simulink library "albedo_lib"  (Simulink 6.3)
undefined symbols (not defined in the file or in its folder): albedo_path, albedo_wrapper, filesep, mean_refl, ss_proj
libraries: simulink x1
settings Model: LastModifiedBy=danji  StrictBusMsg=None

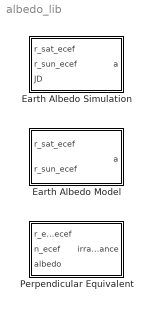
== system albedo_lib ==
  Earth Albedo Model : Subsystem  TreatAsAtomicUnit=on  mask(Earth Albedo Model){refldata=mean_refl, redfac=4, Ts=-1, enable=on}
      mask prompts: refldata "Reflectivity Data (REFL Struct):"; redfac "Reduction factor:"; Ts "Sample Time (-1 for inherited):"
      mask help: Calculcates the Earth albedo from satellite and Sun positions and static reflectivity data.
      mask init:
      | global sy;
      | global sx;
      | sy = floor(180/redfac);
      | sx = floor(288/redfac);
      mask Help:
      | <b>Input</b><br>
      | Sat: Vector to satellite in ECEF [m].<br>
      | Sun: Vector to the Sun in ECEF [m].<p>
      | <b>Parameters</b><br>
      | Reflectivity Data (REFL Struct): TOMS Reflectivity data [E.U].<br>
      | Reduction factor: Reduce data resolution by this factor.<br>
      | Sample Time (-1 for inherited): Sample Time [s]. The block cannot inherit continuous sample time.<br>
      | Enable: Enable or disable albedo calculation.<p>
      | <b>Output</b><br>
      | Albedo: Fraction of solar irradiance received on the satellite. The incoming solar irradiance is 1366.5 W/m^2.<p>
      mask CallbackString: |||enable = strcmp(get_param(gcb,'enable'),'on');
      mask Display:
      | image(imread('private/albedoicon.png'));
      | port_label('output', 1, 'Albedo');
      | port_label('input', 1, 'Sat');
      | port_label('input', 2, 'Sun');
  Earth Albedo Simulation : Subsystem  TreatAsAtomicUnit=on  mask(Earth Albedo Simuation){pathstr=[albedo_path filesep 'refl_data'], redfac=4, Ts=-1, enable=on}
      mask prompts: pathstr "Path to reflectivity data directories:"; redfac "Reduction factor:"; Ts "Sample Time (-1 for inherited):"
      mask help: Calculcates the Earth albedo from satellite and Sun positions and time. The time input is used to search the reflecitivity library for daile reflectivity data.
      mask init:
      | global sy;
      | global sx;
      | sy = floor(180/redfac);
      | sx = floor(288/redfac);
      mask Help:
      | <b>Input</b><br>
      | Sat: Vector to satellite in ECEF [m].<br>
      | Sun: Vector to the Sun in ECEF [m].<br>
      | Time: Time in Julian Date [days].<p>
      | <b>Parameters</b><br>
      | Path to reflectivity data directories: System path to TOMS Earth Reflectivity Data. The data must be structured in i directiry for each year. The path is searched for the newest data, determined from the Time input.<br>
      | Reduction factor: Reduce data resolution by this factor.<br>
      | Sample Time (-1 for inherited): Sample Time [s]. The block cannot inherit continuous sample time.<br>
      | Enable: Enable or disable albedo calculation.<p>
      | <b>Output</b><br>
      | Albedo: Fraction of solar irradiance received on the satellite. The incoming solar irradiance is 1366.5 W/m^2.<p>
      mask CallbackString: |||enable = strcmp(get_param(gcb,'enable'),'on');
      mask Display:
      | image(imread('private/albedoicon.png'));
      | port_label('output', 1, 'Albedo');
      | port_label('input', 1, 'Sat');
      | port_label('input', 2, 'Sun');
      | port_label('input', 3, 'Time');
  Perpendicular Equivalent : Subsystem  mask(Perpendicular Equivalent){Ts=-1, enable=on}
      mask prompts: Ts "Sample Time (-1 for inherited)"
      mask help: Projects all incoming Earth albedo irradiances onto a normal to the exposed surface. The scalar result is the norm of an equivalent perpendicular incident irradiance.
      mask Help:
      | <b>Input</b><br>
      | Nadir: Vector from satellite position to Earth center in ECEF [m].<br>
      | Nss:: Normal vector of exposed surface in ECEF.<br>
      | Albedo: Earth albedo matrix.<p>
      | <b>Parameters</b><br>
      | Sample Time (-1 for inherited): Sample Time [s]. The block cannot inherit continuous sample time.<br>
      | Enable: Enable or disable albedo calculation<p>
      | <b>Output</b><br>
      | IRad: Norm of equivalent incident irradiance vector [W/m^2].<p>
      mask Display:
      | image(imread('private/projectionicon.png'));
      | port_label('output', 1, 'IRad');
      | port_label('input', 1, 'Nadir');
      | port_label('input', 2, 'Nss');
      | port_label('input', 3, 'Albedo');

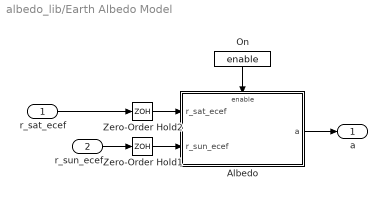
== system albedo_lib/Earth Albedo Model ==
  r_sat_ecef : Inport  SampleTime=Ts
  r_sun_ecef : Inport  Port=2  SampleTime=Ts
  Albedo : Subsystem
  On : Constant  Orientation=down  Value=enable
  Zero-Order Hold1 : ZeroOrderHold  SampleTime=Ts
  Zero-Order Hold2 : ZeroOrderHold  SampleTime=Ts
  a : Outport
  wires:
  On/1 -> Albedo/Enable
  r_sat_ecef/1 -> Zero-Order Hold2/1
  Albedo/1(a) -> a/1
  r_sun_ecef/1 -> Zero-Order Hold1/1
  Zero-Order Hold2/1 -> Albedo/1(r_sat_ecef)
  Zero-Order Hold1/1 -> Albedo/2(r_sun_ecef)

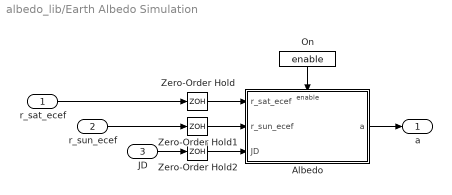
== system albedo_lib/Earth Albedo Simulation ==
  r_sat_ecef : Inport  PortDimensions=3  SampleTime=Ts
  r_sun_ecef : Inport  Port=2  PortDimensions=3  SampleTime=Ts
  JD : Inport  Port=3  PortDimensions=1  SampleTime=Ts
  Albedo : Subsystem
  On : Constant  Orientation=down  Value=enable
  Zero-Order Hold : ZeroOrderHold  SampleTime=Ts
  Zero-Order Hold1 : ZeroOrderHold  SampleTime=Ts
  Zero-Order Hold2 : ZeroOrderHold  SampleTime=Ts
  a : Outport
  wires:
  r_sun_ecef/1 -> Zero-Order Hold1/1
  Albedo/1(a) -> a/1
  r_sat_ecef/1 -> Zero-Order Hold/1
  On/1 -> Albedo/Enable
  JD/1 -> Zero-Order Hold2/1
  Zero-Order Hold/1 -> Albedo/1(r_sat_ecef)
  Zero-Order Hold1/1 -> Albedo/2(r_sun_ecef)
  Zero-Order Hold2/1 -> Albedo/3(JD)

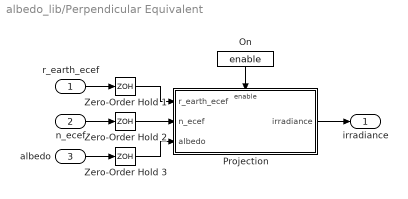
== system albedo_lib/Perpendicular Equivalent ==
  r_earth_ecef : Inport  PortDimensions=3  SampleTime=Ts
  n_ecef : Inport  Port=2  PortDimensions=3  SampleTime=Ts
  albedo : Inport  Port=3  SampleTime=Ts
  On : Constant  Orientation=down  Value=enable
  Projection : Subsystem  TreatAsAtomicUnit=on
  Zero-Order Hold 1 : ZeroOrderHold  SampleTime=Ts
  Zero-Order Hold 2 : ZeroOrderHold  SampleTime=Ts
  Zero-Order Hold 3 : ZeroOrderHold  SampleTime=Ts
  irradiance : Outport  PortDimensions=1  SampleTime=Ts
  wires:
  r_earth_ecef/1 -> Zero-Order Hold 1/1
  n_ecef/1 -> Zero-Order Hold 2/1
  Projection/1(irradiance) -> irradiance/1
  albedo/1 -> Zero-Order Hold 3/1
  Zero-Order Hold 1/1 -> Projection/1(r_earth_ecef)
  Zero-Order Hold 2/1 -> Projection/2(n_ecef)
  Zero-Order Hold 3/1 -> Projection/3(albedo)
  On/1 -> Projection/Enable

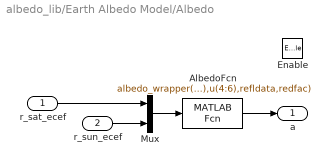
== system albedo_lib/Earth Albedo Model/Albedo ==
  r_sat_ecef : Inport  PortDimensions=3
  r_sun_ecef : Inport  Port=2  PortDimensions=3
  Enable : EnablePort  StatesWhenEnabling=reset
  AlbedoFcn : MATLABFcn  MATLABFcn=albedo_wrapper(u(1:3),u(4:6),refldata,redfac)  OutputDimensions=[sy sx]  OutputSignalType=real  Output1D=off
  Mux : Mux  Inputs=2
  a : Outport  OutputWhenDisabled=reset  InitialOutput=0
  wires:
  r_sun_ecef/1 -> Mux/2
  AlbedoFcn/1 -> a/1
  r_sat_ecef/1 -> Mux/1
  Mux/1 -> AlbedoFcn/1

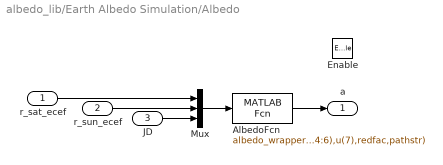
== system albedo_lib/Earth Albedo Simulation/Albedo ==
  r_sat_ecef : Inport  PortDimensions=3
  r_sun_ecef : Inport  Port=2  PortDimensions=3
  JD : Inport  Port=3  PortDimensions=1
  Enable : EnablePort  StatesWhenEnabling=reset
  AlbedoFcn : MATLABFcn  MATLABFcn=albedo_wrapper(u(1:3),u(4:6),u(7),redfac,pathstr)  OutputDimensions=[sy sx]  OutputSignalType=real  Output1D=off
  Mux : Mux  Inputs=3
  a : Outport  OutputWhenDisabled=reset  InitialOutput=0
  wires:
  Mux/1 -> AlbedoFcn/1
  r_sat_ecef/1 -> Mux/1
  AlbedoFcn/1 -> a/1
  r_sun_ecef/1 -> Mux/2
  JD/1 -> Mux/3

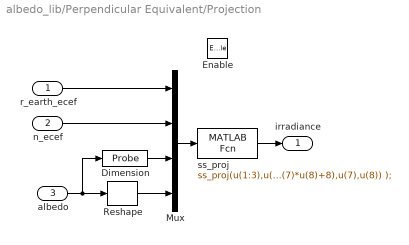
== system albedo_lib/Perpendicular Equivalent/Projection ==
  r_earth_ecef : Inport
  n_ecef : Inport  Port=2
  albedo : Inport  Port=3
  Enable : EnablePort
  Dimension : Probe  ProbeWidth=off  ProbeSampleTime=off  ProbeComplexSignal=off  ProbeSignalDimensions=on
  Mux : Mux
  Reshape : simulink/Math Operations/Reshape  OutputDimensionality=1-D array  OutputDimensions=[1,1]
  ss_proj : MATLABFcn  MATLABFcn=ss_proj(u(1:3),u(4:6),reshape(u(9:u(7)*u(8)+8),u(7),u(8)) );  OutputDimensions=1
  irradiance : Outport
  wires:
  Mux/1 -> ss_proj/1
  r_earth_ecef/1 -> Mux/1
  n_ecef/1 -> Mux/2
  ss_proj/1 -> irradiance/1
  albedo/1 -> Reshape/1, Dimension/1
  Dimension/1 -> Mux/3
  Reshape/1 -> Mux/4
